simulink model "object_tracker_2"  (Simulink 6.4)
settings: Solver=FixedStepDiscrete  StartTime=0.0  StopTime=inf  RelTol=1e-3
model workspace: external: M-Code (data not in the file)
undefined symbols (not defined in the file or in its folder): Kanade, line_row, Lucas, Rec, SDTV
libraries: dspmtrx3 x8, vipsnks x4, viptextngfix x3, dspindex x2, simulink x2, vipconversions x1, dspwin32 x1, vipanalysis x1, vipstatistics x1, vipmisc x1
settings Model: Creator=don  LastModifiedBy=usman  ExtModeAutoUpdateStatusClock=off
settings DataIOCC: LimitDataPoints=off  SaveOutput=off  SignalLogging=off  SaveTime=off  SignalLoggingName=sigsOut
settings OptimizationCC: BufferReusableBoundary=off
settings DebuggingCC: AlgebraicLoopMsg=none  CheckExecutionContextPreStartOutputMsg=on  CheckExecutionContextRuntimeOutputMsg=on  SolverPrmCheckMsg=none  SigSpecEnsureSampleTimeMsg=none  ParameterPrecisionLossMsg=none  BusObjectLabelMismatch=none  StrictBusMsg=None
settings HardwareCC: TargetHWDeviceType=32-bit Generic  ProdEqTarget=off

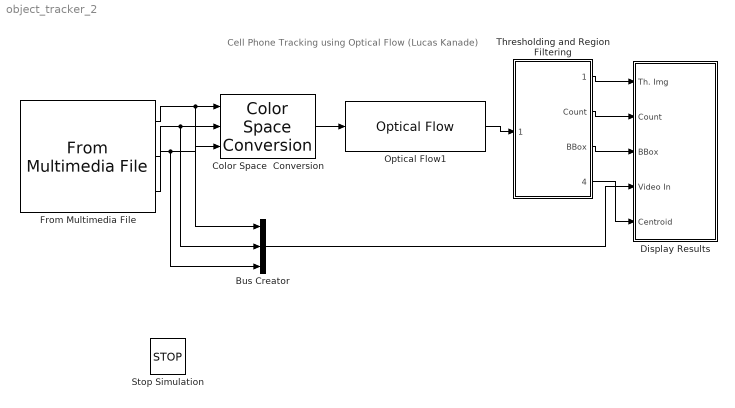
== system object_tracker_2 ==
  note: Cell Phone Tracking using Optical Flow (Lucas Kanade)
  Bus Creator : BusCreator  Inputs=3
  Color Space  Conversion : vipconversions/Color Space  Conversion  conversion=R'G'B' to intensity  wp_str=D65  rec=Rec. 601 (SDTV)  sys=1125/60/2:1
  Display Results : Subsystem
  From Multimedia File : dspwin32/From Multimedia File  DialogController=dspDDGCreate  DialogControllerArgs=DataTag2  inputFilename=C:\fypthings\assorted stuff\whiz\MVI_1730.AVI  loop=on  numPlays=inf  outputStreams=Video only  videoDataType=double  audioDataType=int16  inheritSampleTime=on  userDefinedSampleTime=1/30  noAudioOutput=off  isIntensityVideo=off  outputEOF=off
  Optical Flow1 : vipanalysis/Optical Flow  SystemSampleTime=-1  method=Lucas-Kanade  which2img=Current frame and N-th frame back  N=1  outVelForm=Magnitude-squared  lambda=1  stop_criteria=When maximum number of iterations is reached  maxAllowAbsDiff=eps  maxIter=10  eigTh=0.01
  Stop Simulation : Stop
  Thresholding and Region Filtering : Subsystem
  wires:
  Thresholding and Region Filtering/3(BBox) -> Display Results/3(BBox)
  Thresholding and Region Filtering/2(Count) -> Display Results/2(Count)
  Optical Flow1/1 -> Thresholding and Region Filtering/1(Sq. Mag)
  Color Space  Conversion/1 -> Optical Flow1/1
  Bus Creator/1 -> Display Results/4(Video In)
  Thresholding and Region Filtering/1(Th. Img) -> Display Results/1(Th. Img)
  Thresholding and Region Filtering/4(Centroid) -> Display Results/5(Centroid)
  From Multimedia File/1 -> Color Space  Conversion/1, Bus Creator/1
  From Multimedia File/2 -> Color Space  Conversion/2, Bus Creator/2
  From Multimedia File/3 -> Color Space  Conversion/3, Bus Creator/3

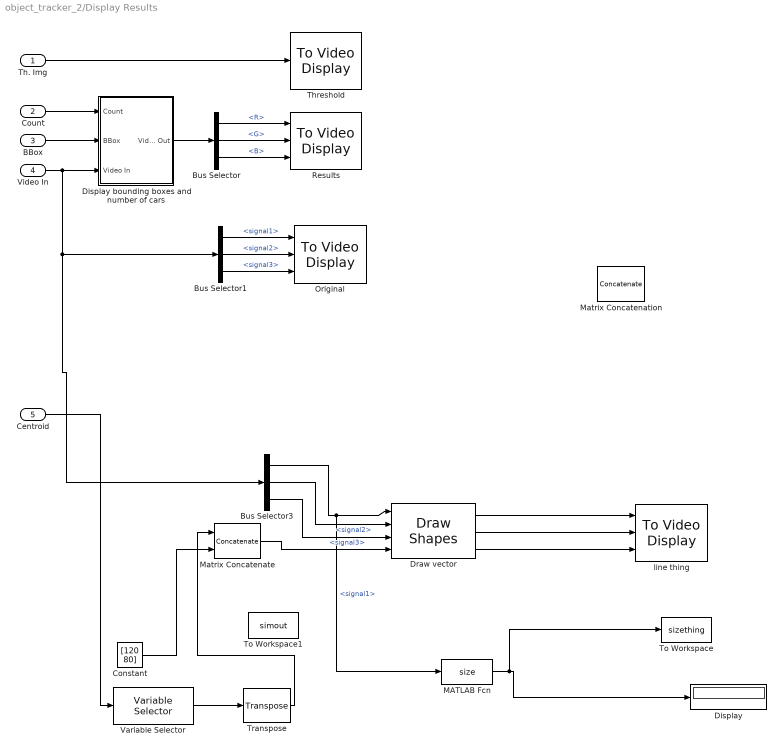
== system object_tracker_2/Display Results ==
  Th. Img : Inport
  Count : Inport  Port=2
  BBox : Inport  Port=3
  Video In : Inport  Port=4
  Centroid : Inport  Port=5
  Bus Selector : BusSelector  OutputSignals=R,G,B
  Bus Selector1 : BusSelector  OutputSignals=signal1,signal2,signal3
  Bus Selector3 : BusSelector  OutputSignals=signal1,signal2,signal3
  Constant : Constant  Value=[120 80]  VectorParams1D=off  OutDataType=sfix(16)  ConRadixGroup=Use specified scaling  OutScaling=2^0  SampleTime=inf  FramePeriod=inf
  Display : Display
  Display bounding boxes and number of cars : Subsystem
  Draw vector : viptextngfix/Draw Shapes  DialogController=vipDDGCreate  DialogControllerArgs=DataTag1  inType=RGB  shape=Lines  fill=off  display=White  intensity=200  color=[200 255 100]  opacity=0.6  viewport=Entire image  antialiasing=off
  MATLAB Fcn : MATLABFcn  MATLABFcn=size  OutputDimensions=[1 2]  Output1D=off
  Matrix Concatenate : Concatenate  Mode=Horizontal matrix concatenation
  Matrix Concatenation : Concatenate  Mode=Horizontal matrix concatenation
  Original : vipsnks/To Video Display  inputType=RGB  OutputDevice=On-screen video monitor  fullScreen=off  videoWindowX=-32000  videoWindowY=-32002  saveWindowSize=off  videoWindowWidth=168  videoWindowHeight=150
  Results : vipsnks/To Video Display  inputType=RGB  OutputDevice=On-screen video monitor  fullScreen=off  videoWindowX=334  videoWindowY=246  saveWindowSize=off  videoWindowWidth=168  videoWindowHeight=150
  Threshold : vipsnks/To Video Display  inputType=Intensity  OutputDevice=On-screen video monitor  fullScreen=off  videoWindowX=-32000  videoWindowY=-32002  saveWindowSize=off  videoWindowWidth=168  videoWindowHeight=150
  To Workspace : ToWorkspace  VariableName=sizething  SampleTime=-1  SaveFormat=Array
  To Workspace1 : ToWorkspace  VariableName=simout  SampleTime=-1  SaveFormat=Structure
  Transpose : dspmtrx3/Transpose  SystemSampleTime=-1  Hermitian=off  overflowFlag=off
  Variable Selector : dspindex/Variable Selector  NumInputs=1  rowsOrCols=Columns  IdxMode=Fixed  Elements=[0]  ZerOneIdxMode=Zero-based  errmode=Clip Index  FillMode=on  FillValues=-1
  line thing : vipsnks/To Video Display  inputType=RGB  OutputDevice=On-screen video monitor  fullScreen=off  videoWindowX=168  videoWindowY=245  saveWindowSize=off  videoWindowWidth=168  videoWindowHeight=150
  wires:
  Video In/1 -> Display bounding boxes and number of cars/3(Video In), Bus Selector1/1, Bus Selector3/1
  Bus Selector/1 -> Results/1  "<R>"
  Bus Selector/2 -> Results/2  "<G>"
  Bus Selector/3 -> Results/3  "<B>"
  Display bounding boxes and number of cars/1(Video Out) -> Bus Selector/1
  Bus Selector1/1 -> Original/1  "<signal1>"
  Bus Selector1/2 -> Original/2  "<signal2>"
  Bus Selector1/3 -> Original/3  "<signal3>"
  Th. Img/1 -> Threshold/1
  Count/1 -> Display bounding boxes and number of cars/1(Count)
  BBox/1 -> Display bounding boxes and number of cars/2(BBox)
  Centroid/1 -> Variable Selector/1
  Constant/1 -> Matrix Concatenate/2
  Matrix Concatenate/1 -> Draw vector/4
  Bus Selector3/1 -> Draw vector/1, MATLAB Fcn/1  "<signal1>"
  Bus Selector3/2 -> Draw vector/2  "<signal2>"
  Bus Selector3/3 -> Draw vector/3  "<signal3>"
  Draw vector/1 -> line thing/1
  Draw vector/2 -> line thing/2
  Draw vector/3 -> line thing/3
  MATLAB Fcn/1 -> Display/1, To Workspace/1
  Transpose/1 -> Matrix Concatenate/1
  Variable Selector/1 -> Transpose/1

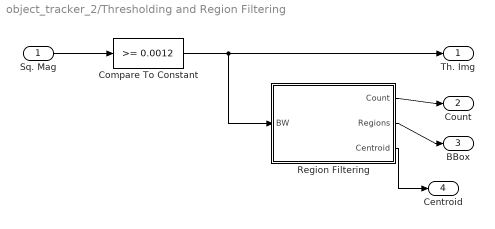
== system object_tracker_2/Thresholding and Region Filtering ==
  Sq. Mag : Inport
  Compare To Constant : simulink/Logic and Bit Operations/Compare To Constant  SystemSampleTime=-1  relop=>=  const=0.0012  LogicOutDataTypeMode=boolean  ZeroCross=off
  Region Filtering : Subsystem
  Th. Img : Outport
  Count : Outport  Port=2
  BBox : Outport  Port=3
  Centroid : Outport  Port=4
  wires:
  Compare To Constant/1 -> Region Filtering/1(BW), Th. Img/1
  Sq. Mag/1 -> Compare To Constant/1
  Region Filtering/1(Count) -> Count/1
  Region Filtering/2(Regions) -> BBox/1
  Region Filtering/3(Centroid) -> Centroid/1

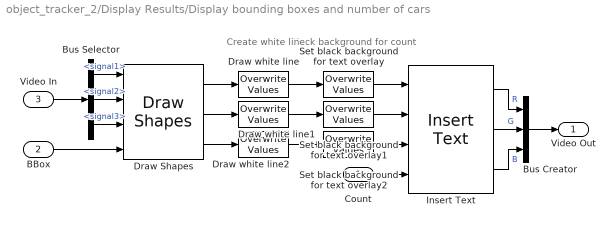
== system object_tracker_2/Display Results/Display bounding boxes and number of cars ==
  note: Black background
      | for count
  note: Create white
      | line
  Count : Inport
  BBox : Inport  Port=2
  Video In : Inport  Port=3
  Bus Creator : BusCreator  Inputs=3
  Bus Selector : BusSelector  OutputSignals=signal1,signal2,signal3
  Draw Shapes : viptextngfix/Draw Shapes  DialogController=vipDDGCreate  DialogControllerArgs=DataTag0  inType=RGB  shape=Rectangles  fill=off  display=User-specified value  intensity=200  color=[0 1 0]  opacity=0.6  viewport=Entire image  antialiasing=off
  Draw white line : dspmtrx3/Overwrite Values  OverWriteDiag=Submatrix  valFrom2ndIP=Specify via dialog  ConstValue=1  RowSpan=Range of rows  RowStartMode=Index  RowStartIndex=22  RowEndMode=Index  RowEndIndex=22+1  ColSpan=All columns  ColStartMode=First  ColStartIndex=1  ColEndMode=Last  ColEndIndex=1  DiagSpan=Range of elements  DiagStartMode=Index  DiagStartIndex=2  DiagEndMode=Index  DiagEndIndex=4
  Draw white line1 : dspmtrx3/Overwrite Values  OverWriteDiag=Submatrix  valFrom2ndIP=Specify via dialog  ConstValue=1  RowSpan=Range of rows  RowStartMode=Index  RowStartIndex=22  RowEndMode=Index  RowEndIndex=22+1  ColSpan=All columns  ColStartMode=First  ColStartIndex=1  ColEndMode=Last  ColEndIndex=1  DiagSpan=Range of elements  DiagStartMode=Index  DiagStartIndex=2  DiagEndMode=Index  DiagEndIndex=4
  Draw white line2 : dspmtrx3/Overwrite Values  OverWriteDiag=Submatrix  valFrom2ndIP=Specify via dialog  ConstValue=1  RowSpan=Range of rows  RowStartMode=Index  RowStartIndex=22  RowEndMode=Index  RowEndIndex=22+1  ColSpan=All columns  ColStartMode=First  ColStartIndex=1  ColEndMode=Last  ColEndIndex=1  DiagSpan=Range of elements  DiagStartMode=Index  DiagStartIndex=2  DiagEndMode=Index  DiagEndIndex=4
  Insert Text : viptextngfix/Insert Text  inputType=RGB  theText='%4d'  fontFace=Arial  dummyVar1=0  blockFontSize=12  antiAliased=on  getTextLocFrom=Specify via dialog  textLoc=[0 0]  getTextColorFrom=Specify via dialog  textColor=[1 1 1]  getTextIntensityFrom=Specify via dialog  textIntensity=1  getTextOpacityFrom=Specify via dialog  textOpacity=1.0  dummyVar2=0  dummyVar3=0  dummyVar4=0
  Set black background for text overlay : dspmtrx3/Overwrite Values  OverWriteDiag=Submatrix  valFrom2ndIP=Specify via dialog  ConstValue=0  RowSpan=Range of rows  RowStartMode=First  RowStartIndex=25  RowEndMode=Index  RowEndIndex=15  ColSpan=Range of columns  ColStartMode=First  ColStartIndex=1  ColEndMode=Index  ColEndIndex=30  DiagSpan=Range of elements  DiagStartMode=Index  DiagStartIndex=2  DiagEndMode=Index  DiagEndIndex=4
  Set black background for text overlay1 : dspmtrx3/Overwrite Values  OverWriteDiag=Submatrix  valFrom2ndIP=Specify via dialog  ConstValue=0  RowSpan=Range of rows  RowStartMode=First  RowStartIndex=25  RowEndMode=Index  RowEndIndex=15  ColSpan=Range of columns  ColStartMode=First  ColStartIndex=1  ColEndMode=Index  ColEndIndex=30  DiagSpan=Range of elements  DiagStartMode=Index  DiagStartIndex=2  DiagEndMode=Index  DiagEndIndex=4
  Set black background for text overlay2 : dspmtrx3/Overwrite Values  OverWriteDiag=Submatrix  valFrom2ndIP=Specify via dialog  ConstValue=0  RowSpan=Range of rows  RowStartMode=First  RowStartIndex=25  RowEndMode=Index  RowEndIndex=15  ColSpan=Range of columns  ColStartMode=First  ColStartIndex=1  ColEndMode=Index  ColEndIndex=30  DiagSpan=Range of elements  DiagStartMode=Index  DiagStartIndex=2  DiagEndMode=Index  DiagEndIndex=4
  Video Out : Outport
  wires:
  Bus Creator/1 -> Video Out/1
  Insert Text/3 -> Bus Creator/3  "B"
  Insert Text/2 -> Bus Creator/2  "G"
  Insert Text/1 -> Bus Creator/1  "R"
  Set black background for text overlay2/1 -> Insert Text/3
  Set black background for text overlay1/1 -> Insert Text/2
  Draw Shapes/3 -> Draw white line2/1
  Draw Shapes/2 -> Draw white line1/1
  Draw white line2/1 -> Set black background for text overlay2/1
  Draw white line1/1 -> Set black background for text overlay1/1
  Count/1 -> Insert Text/4
  Bus Selector/3 -> Draw Shapes/3  "<signal3>"
  Bus Selector/2 -> Draw Shapes/2  "<signal2>"
  Bus Selector/1 -> Draw Shapes/1  "<signal1>"
  Video In/1 -> Bus Selector/1
  BBox/1 -> Draw Shapes/4
  Draw Shapes/1 -> Draw white line/1
  Draw white line/1 -> Set black background for text overlay/1
  Set black background for text overlay/1 -> Insert Text/1

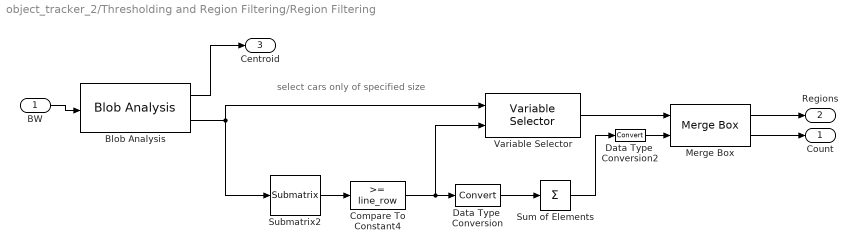
== system object_tracker_2/Thresholding and Region Filtering/Region Filtering ==
  note: select cars only of specified size
  BW : Inport
  Blob Analysis : vipstatistics/Blob Analysis  DialogController=vipDDGCreate  DialogControllerArgs=DataTag3  area=off  centroid=on  bBox=on  majorAxis=off  minorAxis=off  angle=off  eccentricity=off  equivDiameterSq=off  extent=off  perimeter=off  maxBlobs=80  warnIfNumBlobsExceeded=on  isCount=off  useMinArea=on  minArea=200  useMaxArea=on  maxArea=2500  excludeBorderBlob=off  outDT=double  isFill=on  fillValues=-1  conn=8  isLabel=off  outputMode=Binary point scaling  outputWordLength=32  outputFracLength=16  firstCoeffMode=Binary point scaling  firstCoeffWordLength=16  firstCoeffFracLength=14  secondCoeffMode=Binary point scaling  secondCoeffWordLength=32  secondCoeffFracLength=16  accumMode=Binary point scaling  accumWordLength=32  accumFracLength=0  prodOutputMode=Binary point scaling  prodOutputWordLength=32  prodOutputFracLength=16  roundingMode=Floor  overflowMode=off
  Compare To Constant4 : simulink/Logic and Bit Operations/Compare To Constant  SystemSampleTime=-1  relop=>=  const=line_row  LogicOutDataTypeMode=boolean  ZeroCross=off
  Data Type  Conversion : DataTypeConversion  OutDataTypeMode=single  SaturateOnIntegerOverflow=on  RndMeth=Zero
  Data Type  Conversion2 : DataTypeConversion  OutDataTypeMode=int32  SaturateOnIntegerOverflow=on  RndMeth=Zero
  Merge Box : vipmisc/Merge Box  whichdir=Row direction only  cdist=60  rdist=45
  Submatrix2 : dspmtrx3/Submatrix  RowSpan=One row  RowStartMode=Index  RowStartIndex=1  RowEndMode=Last  RowEndIndex=1  ColSpan=All columns  ColStartMode=First  ColStartIndex=1  ColEndMode=Last  ColEndIndex=1
  Sum of Elements : Sum  Inputs=+  OutScaling=2^-10
  Variable Selector : dspindex/Variable Selector  NumInputs=1  rowsOrCols=Columns  IdxMode=Variable  Elements=[1 3]  ZerOneIdxMode=Zero-based  errmode=Clip Index  FillMode=on  FillValues=-1
  Count : Outport
  Regions : Outport  Port=2
  Centroid : Outport  Port=3
  wires:
  Data Type  Conversion/1 -> Sum of Elements/1
  Sum of Elements/1 -> Data Type  Conversion2/1
  Compare To Constant4/1 -> Data Type  Conversion/1, Variable Selector/2
  Submatrix2/1 -> Compare To Constant4/1
  BW/1 -> Blob Analysis/1
  Variable Selector/1 -> Merge Box/1
  Merge Box/1 -> Regions/1
  Merge Box/2 -> Count/1
  Data Type  Conversion2/1 -> Merge Box/2
  Blob Analysis/2 -> Submatrix2/1, Variable Selector/1
  Blob Analysis/1 -> Centroid/1
